simulink model "nonlin_unique_plane"  (Simulink 6.0)
settings: Solver=ode45  StartTime=0.0  StopTime=300  RelTol=1e-3
undefined symbols (not defined in the file): B, DQ, DQL, I, m, M, Ma, MaU, rg, T, W, xb, xg, Xudot, yb, yg, Yvdot, zb, zg, Zwdot
libraries: simulink x24, rov_design_analysis x16
(part 3 of 3)

== system nonlin_unique_plane/Open-loop  ROV System1/Euler Transformation  /Transformation matrix T/Row2 of R ==
  translational body velocity : Inport  Port=1  LatchInput=off
  angular position : Inport  Port=2  LatchInput=off
  -cZ.sX+sY.sZ.cX : Fcn  Expr=-cos(u[3])*sin(u[1]) + sin(u[2])*sin(u[3])*cos(u[1])
  Dot Product1 : simulink/Math Operations/Dot Product  InputSameDT=on  OutDataType=sfix(16)  OutScaling=2^-10  DoSatur=off
  Mux1 : Mux  Inputs=3
  cY.sZ : Fcn  Expr=sin(u[3]) * cos(u[2])
  cZ.cX+sX.sY.sZ : Fcn  Expr=cos(u[3])*cos(u[1]) + sin(u[1])*sin(u[2])*sin(u[3])
  translational earth velocity (row 2) : Outport
  wires:
  Dot Product1/1 -> translational earth velocity (row 2)/1
  translational body velocity/1 -> Dot Product1/2
  Mux1/1 -> Dot Product1/1
  -cZ.sX+sY.sZ.cX/1 -> Mux1/3
  cZ.cX+sX.sY.sZ/1 -> Mux1/2
  cY.sZ/1 -> Mux1/1
  angular position/1 -> -cZ.sX+sY.sZ.cX/1, cZ.cX+sX.sY.sZ/1, cY.sZ/1

== system nonlin_unique_plane/Open-loop  ROV System1/Euler Transformation  /Transformation matrix T/Row3 of R ==
  translational body velocity : Inport  Port=1  LatchInput=off
  angular position : Inport  Port=2  LatchInput=off
  -sY : Fcn  Expr=-sin(u[2])
  Dot Product1 : simulink/Math Operations/Dot Product  InputSameDT=on  OutDataType=sfix(16)  OutScaling=2^-10  DoSatur=off
  Mux1 : Mux  Inputs=3
  cY.cX : Fcn  Expr=cos(u[2])*cos(u[1])
  cY.sX : Fcn  Expr=cos(u[2])*sin(u[1])
  translational earth velocity (row 3) : Outport  InitialOutput=0
  wires:
  Dot Product1/1 -> translational earth velocity (row 3)/1
  translational body velocity/1 -> Dot Product1/2
  Mux1/1 -> Dot Product1/1
  cY.cX/1 -> Mux1/3
  cY.sX/1 -> Mux1/2
  -sY/1 -> Mux1/1
  angular position/1 -> cY.cX/1, cY.sX/1, -sY/1
